simulink model "model2g"  (R2020a)
settings: Solver=VariableStepAuto  StartTime=0.0  StopTime=10.0  RelTol=1e-3
values from neighbouring files (symbols this model uses):
  A = [ ... (first row only)    [a2p1.m]    (also in p1.m; p2f.m; p2g.m)
  B = [0; 0; 0; 0; 7.5]    [p2f.m]    (also in p2g.m = [0; 0; 0; 0; 7.5;])
  C = [ 1 0 0 0 0 ... (first row only)    [p2f.m]    (also in p2g.m)
  g = 9.81    [a2p2.m]    (also in p2c_e.m; p2f.m; p2g.m)
  k_intwind = kp_phi*kp_chi*0.5    [p2g.m]
  kd_phi = (2*zeta_phi*omega_n_phi - a_phi1)/a_phi2    [a2p2.m]    (also in p2c.m = 2.24; p2c_e.m; p2f.m; p2g.m)
  ki_chi = (omega_n_chi)^2 * V_g/g    [a2p2.m]    (also in p2c_e.m; p2f.m; p2g.m)
  kp_chi = 2*zeta_chi*omega_n_chi*V_g/g    [a2p2.m]    (also in p2c_e.m; p2f.m; p2g.m)
  kp_phi = (delta_max_a/e_max_a)*sign(a_phi2)    [a2p2.m]    (also in p2c.m = delta_max / e_phimax * sign(a_phi2); p2c_e.m; p2f.m; p2g.m)
  V_g = V_a    (= 580)    [a2p2.m]    (also in p2c_e.m; p2f.m; p2g.m)
libraries: simulink_extras x3
settings Model: Creator=ivermyklebust  LastModifiedBy=ivermyklebust

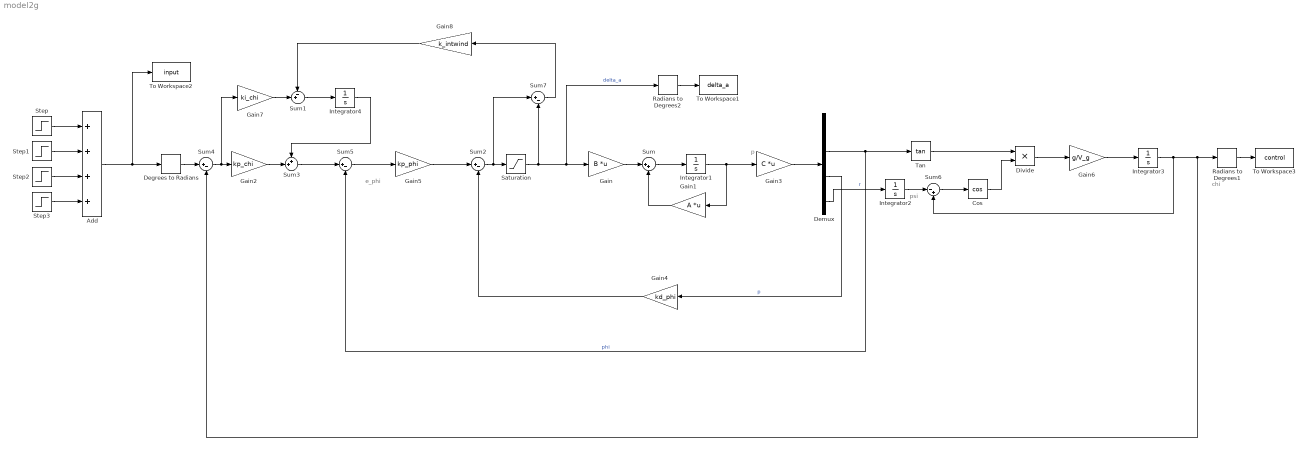
== system model2g ==
  note: p
  note: psi
  note: e_phi
  note: chi
  Add : Sum  Inputs=++++
  Cos : Trigonometry  Operator=cos
  Degrees to Radians : simulink_extras/Transformations/Degrees to Radians
  Demux : Demux
  Divide : Product  Inputs=**
  Gain : Gain  Gain=B  Multiplication=Matrix(K*u)
  Gain1 : Gain  Gain=A  Multiplication=Matrix(K*u)
  Gain2 : Gain  Gain=kp_chi
  Gain3 : Gain  Gain=C  Multiplication=Matrix(K*u)
  Gain4 : Gain  Gain=kd_phi
  Gain5 : Gain  Gain=kp_phi
  Gain6 : Gain  Gain=g/V_g
  Gain7 : Gain  Gain=ki_chi
  Gain8 : Gain  Gain=k_intwind
  Integrator{1..4} (4 alike) : Integrator
  Radians to Degrees1 : simulink_extras/Transformations/Radians to Degrees
  Radians to Degrees2 : simulink_extras/Transformations/Radians to Degrees
  Saturation : Saturate  UpperLimit=pi/6  LowerLimit=-pi/6
  Step : Step  Time=100  After=7.5  SampleTime=0
  Step1 : Step  Time=200  After=7.5  SampleTime=0
  Step2 : Step  Time=300  After=-7.5  SampleTime=0
  Step3 : Step  Time=400  After=0  SampleTime=0
  Sum : Sum  Inputs=|++
  Sum1 : Sum  Inputs=-+|
  Sum{2,4..5,7} (4 alike) : Sum  Inputs=|+-
  Sum3 : Sum  Inputs=++|
  Sum6 : Sum  Inputs=|-+
  Tan : Trigonometry  Operator=tan
  To Workspace1 : ToWorkspace  VariableName=delta_a  SaveFormat=Timeseries  SampleTime=-1
  To Workspace2 : ToWorkspace  VariableName=input  SaveFormat=Timeseries  SampleTime=-1
  To Workspace3 : ToWorkspace  VariableName=control  SaveFormat=Timeseries  SampleTime=-1
  wires:
  Gain6/1 -> Integrator3/1
  Tan/1 -> Divide/1
  Divide/1 -> Gain6/1
  Integrator4/1 -> Sum3/1
  Integrator2/1 -> Sum6/1
  Step3/1 -> Add/4
  Step/1 -> Add/1
  Integrator1/1 -> Gain3/1, Gain1/1
  Demux/2 -> Tan/1, Sum5/2  "phi"
  Step2/1 -> Add/3
  Gain4/1 -> Sum2/2
  Gain2/1 -> Sum3/2
  Cos/1 -> Divide/2
  Step1/1 -> Add/2
  Gain/1 -> Sum/1
  Sum4/1 -> Gain7/1, Gain2/1
  Sum2/1 -> Sum7/1, Saturation/1
  Gain5/1 -> Sum2/1
  Gain1/1 -> Sum/2
  Radians to Degrees2/1 -> To Workspace1/1
  Degrees to Radians/1 -> Sum4/1
  Demux/3 -> Gain4/1  "p"
  Add/1 -> To Workspace2/1, Degrees to Radians/1
  Saturation/1 -> Radians to Degrees2/1, Gain/1, Sum7/2  "delta_a"
  Sum/1 -> Integrator1/1
  Integrator3/1 -> Sum4/2, Radians to Degrees1/1, Sum6/2
  Sum6/1 -> Cos/1
  Sum3/1 -> Sum5/1
  Gain3/1 -> Demux/1
  Demux/4 -> Integrator2/1  "r"
  Sum5/1 -> Gain5/1
  Radians to Degrees1/1 -> To Workspace3/1
  Gain7/1 -> Sum1/2
  Sum1/1 -> Integrator4/1
  Sum7/1 -> Gain8/1
  Gain8/1 -> Sum1/1
